simulink model "Test2MotorParameters"  (R2023b)
settings: Solver=FixedStepAuto  StartTime=0.0  StopTime=inf  RelTol=1e-3  EnableMultiTasking=on
model workspace (MAT data in the model file):
  Can_ID = 0
  MyCanID = 1
libraries: canmsglib x7, arduinolib x5
settings Model: SimulationMode=external  ExtModeTrigDuration=2  Creator=Antonio  LastModifiedBy=Antonio
settings OptimizationCC: EnhancedBackFolding=on  PassReuseOutputArgsAs=Individual arguments  ZeroExternalMemoryAtStartup=off  ZeroInternalMemoryAtStartup=off  MaxStackSize=64  OptimizeBlockOrder=speed  DifferentSizesBufferReuse=on  OptimizationCustomize=off  EfficientTunableParamExpr=on
settings DebuggingCC: ParameterTunabilityLossMsg=error
settings HardwareCC: ProdBitPerPointer=32  ProdBitPerSizeT=32  ProdBitPerPtrDiffT=32  ProdLargestAtomicInteger=Long  ProdLargestAtomicFloat=Double  ProdWordSize=32  ProdHWDeviceType=ARM Compatible->ARM Cortex
settings SFSimCC: MATLABDynamicMemAlloc=off
settings RTWCC: Description=Embedded Coder  SystemTargetFile=ert.tlc  HardwareBoard=Arduino MKR WiFi 1010  TemplateMakefile=ert_default_tmf  Toolchain=Arduino ARM  BuildConfiguration=Faster Runs
settings CodeAppCC: ForceParamTrailComments=on  IgnoreCustomStorageClasses=off  OperatorAnnotations=on  SimulinkDataObjDesc=on  SFDataObjDesc=on  InsertBlockDesc=on
settings ERTTargetCC: SupportContinuousTime=on  SupportVariableSizeSignals=on  ExtMode=on  ExtModeTransport=3  ExtModeStaticAlloc=on  ExtModeAutomaticAllocSize=off  ExtModeStaticAllocSize=8192  ExtModeMexFile=ext_xcp  ExtModeMexArgs=0 13 921600  ExtModeIntrfLevel=Level2 - Open

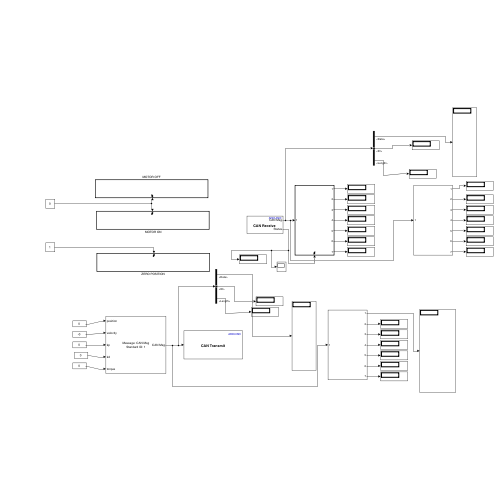
[thumbnail: Simulink's stored preview of the top-level diagram]
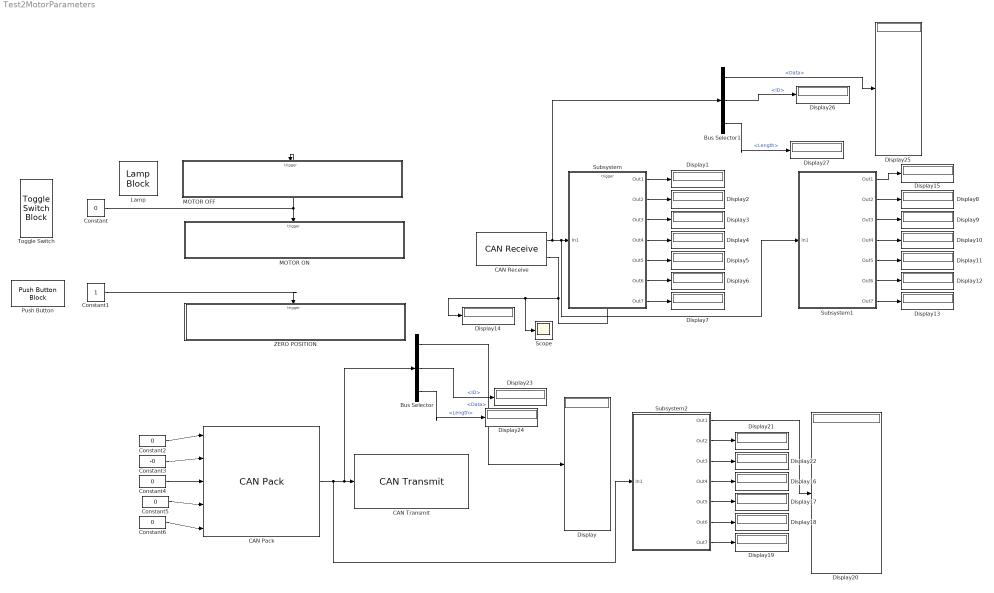
== system Test2MotorParameters ==
  " MOTOR ON" : Subsystem
  Bus Selector : BusSelector  OutputSignals=Data,ID,Length
  Bus Selector1 : BusSelector  OutputSignals=Data,ID,Length
  CAN Pack : canmsglib/CAN Pack  MsgList=(none)  MsgName=CAN Msg  MsgIDType=Standard (11-bit identifier)  MsgIdentifier=1  MsgLength=8  Remote=off  ApplyMinMax=off  BusOutput=on  SignalInfo={ 'position', '8', '16', 'BE', 'signed', 'Standard', '0', '1', '-95.5', '-95.5', '95.5'; 'velocity', '28', '12', 'BE', 'signed', 'Standard', '0', '1', '-45', '-45', '45'; 'kp', '32', '12', 'BE', 'unsigned', 'Standard', '0', '1', '0', '0', '500'; 'kd', '52', '12', 'BE', 'unsigned', 'Standard', '0', '1', '0', '0', '5'; 'torque', '56', '12', 'BE', 'signed', 'Standard', '0', '1', '-18', '-18', '18' }
      settings: LibrarySourceBlock=embeddedtargetslib/Host Communication/CAN Pack  DataFormat=manually specified signals
  CAN Receive : arduinolib/CAN Receive  outputDataType=CAN Msg  identifierType=Standard (11-bit identifier)  messageId=100  msgLength=8  SampleTime=0.01  outputError=off  outputRemote=off
  CAN Transmit : arduinolib/CAN Transmit  inputDataType=CAN Msg  BlockingMode_=on  BlockTimeout_=1  outputStatus=off  identifierType=Standard (11-bit identifier)  messageId=100  msgLength=8  remoteFrame=off
  Constant : Constant  Value=0
  Constant1 : Constant
  Constant{2,4..6} (4 alike) : Constant  Value=0  OutDataTypeStr=single
  Constant3 : Constant  Value=-0  OutDataTypeStr=single
  Display{,1..27} (28 alike) : Display
  Lamp : LampBlock  LabelPosition=Hide
  MOTOR OFF : Subsystem
  Push Button : PushButtonBlock  Icon=AntilockBrakeSystem  OffValue=1.000000
  Scope : Scope
  Subsystem : Subsystem
  Subsystem1 : Subsystem
  Subsystem2 : Subsystem
  Toggle Switch : ToggleSwitchBlock
      settings: Values={{'Off', 'On'}, [0 1]}
  ZERO POSITION : Subsystem
  wires:
  Subsystem/1(Out1) -> Display1/1
  Subsystem/2(Out2) -> Display2/1
  Subsystem/3(Out3) -> Display3/1
  Subsystem/4(Out4) -> Display4/1
  Subsystem/5(Out5) -> Display5/1
  Subsystem/6(Out6) -> Display6/1
  Subsystem/7(Out7) -> Display7/1
  CAN Receive/2 -> Scope/1, Display14/1, Subsystem/Trigger
  Subsystem1/7(Out7) -> Display13/1
  Subsystem1/6(Out6) -> Display12/1
  Subsystem1/5(Out5) -> Display11/1
  Subsystem1/4(Out4) -> Display10/1
  Subsystem1/3(Out3) -> Display9/1
  Subsystem1/2(Out2) -> Display8/1
  Subsystem1/1(Out1) -> Display15/1
  Constant/1 -> " MOTOR ON"/Trigger, MOTOR OFF/Trigger
  Constant1/1 -> ZERO POSITION/Trigger
  Constant2/1 -> CAN Pack/1
  Constant3/1 -> CAN Pack/2
  Constant4/1 -> CAN Pack/3
  Constant5/1 -> CAN Pack/4
  Constant6/1 -> CAN Pack/5
  Subsystem2/1(Out1) -> Display20/1
  Subsystem2/2(Out2) -> Display21/1
  Subsystem2/3(Out3) -> Display22/1
  Subsystem2/4(Out4) -> Display16/1
  Subsystem2/5(Out5) -> Display17/1
  Subsystem2/6(Out6) -> Display18/1
  Subsystem2/7(Out7) -> Display19/1
  CAN Pack/1 -> Subsystem2/1(In1), Bus Selector/1, CAN Transmit/1
  Bus Selector/1 -> Display/1  "<Data>"
  Bus Selector/2 -> Display23/1  "<ID>"
  Bus Selector/3 -> Display24/1  "<Length>"
  Bus Selector1/2 -> Display26/1  "<ID>"
  Bus Selector1/1 -> Display25/1  "<Data>"
  Bus Selector1/3 -> Display27/1  "<Length>"
  CAN Receive/1 -> Bus Selector1/1, Subsystem1/1(In1), Subsystem/1(In1)

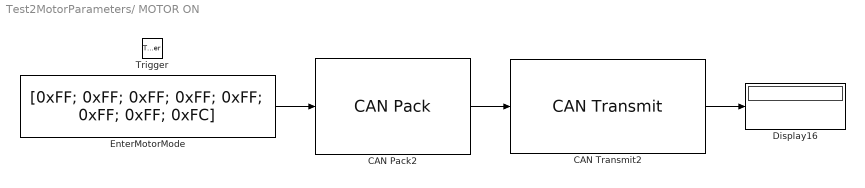
== system Test2MotorParameters/ MOTOR ON ==
  Trigger : TriggerPort  VariantControl=(inherit)  PortDimensions=1
  CAN Pack2 : canmsglib/CAN Pack  MsgList=(none)  MsgName=CAN Msg  MsgIDType=Standard (11-bit identifier)  MsgIdentifier=MyCanID  MsgLength=8  Remote=off  ApplyMinMax=off  BusOutput=on  SignalInfo={ 'position', '8', '16', 'BE', 'signed', 'Standard', '0', '1', '-95.5', '-95.5', '95.5'; 'velocity', '28', '12', 'BE', 'signed', 'Standard', '0', '1', '-45', '-45', '45'; 'kp', '32', '12', 'BE', 'unsigned', 'Standard', '0', '1', '0', '0', '500'; 'kd', '52', '12', 'BE', 'unsigned', 'Standard', '0', '1', '0', '0', '5'; 'torque', '56', '12', 'BE', 'signed', 'Standard', '0', '1', '-18', '-18', '18' }
      settings: LibrarySourceBlock=embeddedtargetslib/Host Communication/CAN Pack  DataFormat=raw data
  CAN Transmit2 : arduinolib/CAN Transmit  inputDataType=CAN Msg  BlockingMode_=on  BlockTimeout_=1  outputStatus=on  identifierType=Standard (11-bit identifier)  messageId=100  msgLength=8  remoteFrame=off
  Display16 : Display
  EnterMotorMode : Constant  Value=|  OutDataTypeStr=uint8
      | [0xFF; 0xFF; 0xFF; 0xFF; 0xFF;
      | 0xFF;
      | 0xFF;
      | 0xFC]
  wires:
  CAN Transmit2/1 -> Display16/1
  EnterMotorMode/1 -> CAN Pack2/1
  CAN Pack2/1 -> CAN Transmit2/1

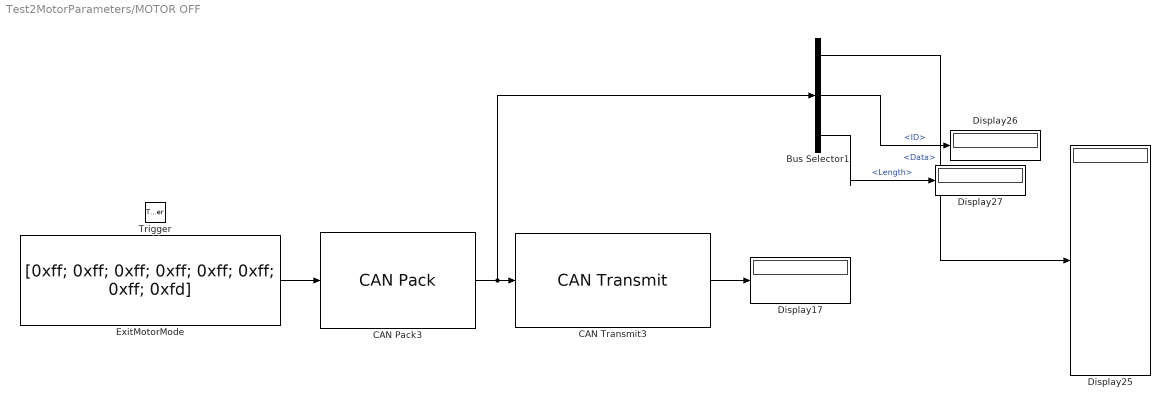
== system Test2MotorParameters/MOTOR OFF ==
  Trigger : TriggerPort  TriggerType=falling  VariantControl=(inherit)  PortDimensions=1
  Bus Selector1 : BusSelector  OutputSignals=Data,ID,Length
  CAN Pack3 : canmsglib/CAN Pack  MsgList=(none)  MsgName=CAN Msg  MsgIDType=Standard (11-bit identifier)  MsgIdentifier=MyCanID  MsgLength=8  Remote=on  ApplyMinMax=off  BusOutput=on  SignalInfo={ 'position', '8', '16', 'BE', 'signed', 'Standard', '0', '1', '-95.5', '-95.5', '95.5'; 'velocity', '28', '12', 'BE', 'signed', 'Standard', '0', '1', '-45', '-45', '45'; 'kp', '32', '12', 'BE', 'unsigned', 'Standard', '0', '1', '0', '0', '500'; 'kd', '52', '12', 'BE', 'unsigned', 'Standard', '0', '1', '0', '0', '5'; 'torque', '56', '12', 'BE', 'signed', 'Standard', '0', '1', '-18', '-18', '18' }
      settings: LibrarySourceBlock=embeddedtargetslib/Host Communication/CAN Pack  DataFormat=raw data
  CAN Transmit3 : arduinolib/CAN Transmit  inputDataType=CAN Msg  BlockingMode_=on  BlockTimeout_=1  outputStatus=on  identifierType=Standard (11-bit identifier)  messageId=100  msgLength=8  remoteFrame=off
  Display{17,25..27} (4 alike) : Display
  ExitMotorMode : Constant  Value=|  OutDataTypeStr=uint8
      | [0xff; 0xff; 0xff; 0xff; 0xff;
      | 0xff;
      | 0xff;
      | 0xfd]
  wires:
  ExitMotorMode/1 -> CAN Pack3/1
  CAN Transmit3/1 -> Display17/1
  Bus Selector1/2 -> Display26/1  "<ID>"
  Bus Selector1/1 -> Display25/1  "<Data>"
  Bus Selector1/3 -> Display27/1  "<Length>"
  CAN Pack3/1 -> Bus Selector1/1, CAN Transmit3/1

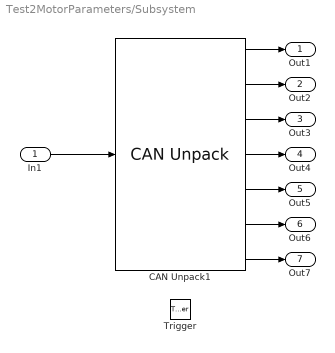
== system Test2MotorParameters/Subsystem ==
  In1 : Inport
  Trigger : TriggerPort  VariantControl=(inherit)  PortDimensions=1
  CAN Unpack1 : canmsglib/CAN Unpack  MsgList=(none)  MsgName=CAN Msg  MsgIDType=Standard (11-bit identifier)  MsgIdentifier=1  MsgLength=5  SignalInfo={ 'position', '8', '16', 'BE', 'signed', 'Standard', '0', '343.11518324607329842931937172775', '-95.5', '-95.5', '95.5'; 'velocity', '28', '12', 'BE', 'signed', 'Standard', '0', '45.5', '-45', '-45', '45'; 'current', '32', '12', 'BE', 'signed', 'Standard', '0', '113.75', '-18', '-18', '18' }  IDPort=on  TimestampPort=on  ErrorPort=on  RemotePort=off  LengthPort=off  StatusPort=on  ApplyMinMax=off
      settings: LibrarySourceBlock=embeddedtargetslib/Host Communication/CAN Unpack
  Out1 : Outport
  Out2 : Outport  Port=2
  Out3 : Outport  Port=3
  Out4 : Outport  Port=4
  Out5 : Outport  Port=5
  Out6 : Outport  Port=6
  Out7 : Outport  Port=7
  wires:
  CAN Unpack1/2 -> Out2/1
  CAN Unpack1/7 -> Out7/1
  In1/1 -> CAN Unpack1/1
  CAN Unpack1/5 -> Out5/1
  CAN Unpack1/4 -> Out4/1
  CAN Unpack1/1 -> Out1/1
  CAN Unpack1/6 -> Out6/1
  CAN Unpack1/3 -> Out3/1

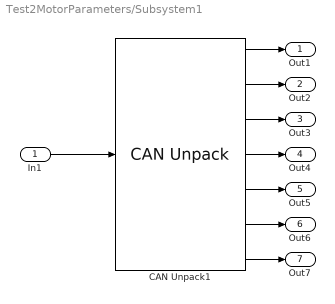
== system Test2MotorParameters/Subsystem1 ==
  In1 : Inport
  CAN Unpack1 : canmsglib/CAN Unpack  MsgList=(none)  MsgName=CAN Msg  MsgIDType=Standard (11-bit identifier)  MsgIdentifier=1  MsgLength=5  SignalInfo={ 'position', '8', '16', 'BE', 'signed', 'Standard', '0', '343.11518324607329842931937172775', '-95.5', '-95.5', '95.5'; 'velocity', '28', '12', 'BE', 'signed', 'Standard', '0', '45.5', '-45', '-45', '45'; 'current', '32', '12', 'BE', 'signed', 'Standard', '0', '113.75', '-18', '-18', '18' }  IDPort=on  TimestampPort=on  ErrorPort=on  RemotePort=off  LengthPort=off  StatusPort=on  ApplyMinMax=off
      settings: LibrarySourceBlock=embeddedtargetslib/Host Communication/CAN Unpack
  Out1 : Outport
  Out2 : Outport  Port=2
  Out3 : Outport  Port=3
  Out4 : Outport  Port=4
  Out5 : Outport  Port=5
  Out6 : Outport  Port=6
  Out7 : Outport  Port=7
  wires:
  CAN Unpack1/3 -> Out3/1
  CAN Unpack1/6 -> Out6/1
  CAN Unpack1/1 -> Out1/1
  CAN Unpack1/4 -> Out4/1
  CAN Unpack1/5 -> Out5/1
  In1/1 -> CAN Unpack1/1
  CAN Unpack1/7 -> Out7/1
  CAN Unpack1/2 -> Out2/1

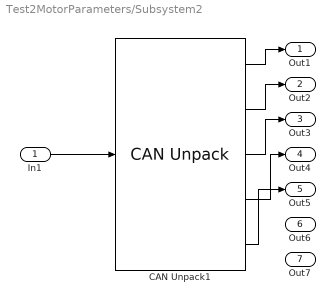
== system Test2MotorParameters/Subsystem2 ==
  In1 : Inport
  CAN Unpack1 : canmsglib/CAN Unpack  MsgList=(none)  MsgName=CAN Msg  MsgIDType=Standard (11-bit identifier)  MsgIdentifier=1  MsgLength=8  SignalInfo={ 'position', '8', '16', 'BE', 'signed', 'Standard', '0', '343.11518324607329842931937172775', '-95.5', '-95.5', '95.5'; 'velocity', '28', '12', 'BE', 'signed', 'Standard', '0', '45.5', '-45', '-45', '45'; 'current', '32', '12', 'BE', 'signed', 'Standard', '0', '113.75', '-18', '-18', '18' }  IDPort=on  TimestampPort=on  ErrorPort=on  RemotePort=off  LengthPort=off  StatusPort=on  ApplyMinMax=off
      settings: LibrarySourceBlock=embeddedtargetslib/Host Communication/CAN Unpack  DataFormat=raw data
  Out1 : Outport
  Out2 : Outport  Port=2
  Out3 : Outport  Port=3
  Out4 : Outport  Port=4
  Out5 : Outport  Port=5
  Out6 : Outport  Port=6
  Out7 : Outport  Port=7
  wires:
  CAN Unpack1/2 -> Out2/1
  ? -> Out7/1
  In1/1 -> CAN Unpack1/1
  CAN Unpack1/5 -> Out5/1
  CAN Unpack1/4 -> Out4/1
  CAN Unpack1/1 -> Out1/1
  ? -> Out6/1
  CAN Unpack1/3 -> Out3/1

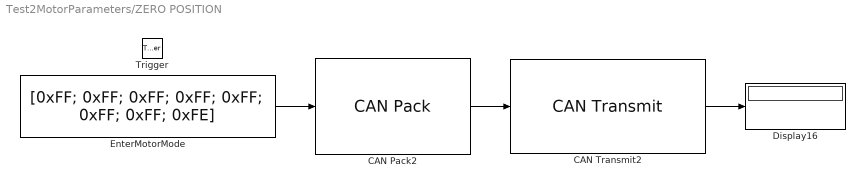
== system Test2MotorParameters/ZERO POSITION ==
  Trigger : TriggerPort  VariantControl=(inherit)  PortDimensions=1
  CAN Pack2 : canmsglib/CAN Pack  MsgList=(none)  MsgName=CAN Msg  MsgIDType=Standard (11-bit identifier)  MsgIdentifier=MyCanID  MsgLength=8  Remote=off  ApplyMinMax=off  BusOutput=on  SignalInfo={ 'position', '8', '16', 'BE', 'signed', 'Standard', '0', '1', '-95.5', '-95.5', '95.5'; 'velocity', '28', '12', 'BE', 'signed', 'Standard', '0', '1', '-45', '-45', '45'; 'kp', '32', '12', 'BE', 'unsigned', 'Standard', '0', '1', '0', '0', '500'; 'kd', '52', '12', 'BE', 'unsigned', 'Standard', '0', '1', '0', '0', '5'; 'torque', '56', '12', 'BE', 'signed', 'Standard', '0', '1', '-18', '-18', '18' }
      settings: LibrarySourceBlock=embeddedtargetslib/Host Communication/CAN Pack  DataFormat=raw data
  CAN Transmit2 : arduinolib/CAN Transmit  inputDataType=CAN Msg  BlockingMode_=on  BlockTimeout_=1  outputStatus=on  identifierType=Standard (11-bit identifier)  messageId=100  msgLength=8  remoteFrame=off
  Display16 : Display
  EnterMotorMode : Constant  Value=|  OutDataTypeStr=uint8
      | [0xFF; 0xFF; 0xFF; 0xFF; 0xFF;
      | 0xFF;
      | 0xFF;
      | 0xFE]
  wires:
  CAN Pack2/1 -> CAN Transmit2/1
  EnterMotorMode/1 -> CAN Pack2/1
  CAN Transmit2/1 -> Display16/1
